simulink model "crossMatrix"  (R2018a)
settings: Solver=VariableStepAuto  StartTime=0.0  StopTime=10.0  RelTol=1e-3
settings Model: Creator=henry  LastModifiedBy=henry

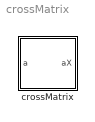
== system crossMatrix ==
  "crossMatrix " : Subsystem  mask(Cross Matrix){}
      mask help: This block takes in a 3x1 vector and outputs it's corresponding 3x3 cross product matrix

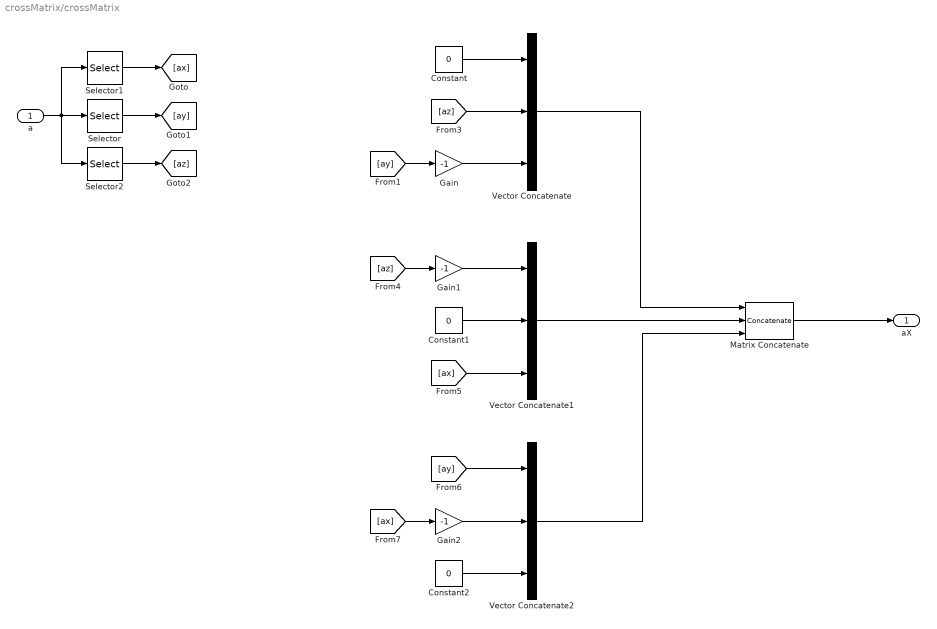
== system crossMatrix/crossMatrix  ==
  a : Inport
  Constant : Constant  Value=0
  Constant1 : Constant  Value=0
  Constant2 : Constant  Value=0
  Gain : Gain  Gain=-1
  Gain1 : Gain  Gain=-1
  Gain2 : Gain  Gain=-1
  Matrix Concatenate : Concatenate  NumInputs=3  Mode=Multidimensional array  ConcatenateDimension=2
  Selector : Selector  InputPortWidth=3  IndexOptions=Index vector (dialog)  Indices=2  OutputSizes=1
  Selector1 : Selector  InputPortWidth=3  IndexOptions=Index vector (dialog)  Indices=1  OutputSizes=1
  Selector2 : Selector  InputPortWidth=3  IndexOptions=Index vector (dialog)  Indices=3  OutputSizes=1
  Vector Concatenate : Concatenate  NumInputs=3
  Vector Concatenate1 : Concatenate  NumInputs=3
  Vector Concatenate2 : Concatenate  NumInputs=3
  aX : Outport
  wires:
  Selector/1 -> [ay]
  a/1 -> Selector2/1, Selector1/1, Selector/1
  Constant/1 -> Vector Concatenate/1
  Gain1/1 -> Vector Concatenate1/1
  [az] -> Vector Concatenate/2
  Selector2/1 -> [az]
  Selector1/1 -> [ax]
  Vector Concatenate/1 -> Matrix Concatenate/1
  Gain/1 -> Vector Concatenate/3
  Vector Concatenate2/1 -> Matrix Concatenate/3
  [ax] -> Gain2/1
  Constant2/1 -> Vector Concatenate2/3
  Matrix Concatenate/1 -> aX/1
  Vector Concatenate1/1 -> Matrix Concatenate/2
  [ay] -> Vector Concatenate2/1
  [ax] -> Vector Concatenate1/3
  Constant1/1 -> Vector Concatenate1/2
  Gain2/1 -> Vector Concatenate2/2
  [az] -> Gain1/1
  [ay] -> Gain/1
